simulink model "V2_Modell_RLC"  (R2022a)
settings: Solver=ode3  StartTime=0.0  StopTime=Zeit(end)  FixedStep=0.000001  RelTol=1e-3
values from neighbouring files (symbols this model uses):
  den = [(C*L*R_d*R_v) (R_d*L + R_v*L + R_v*R_d*R_L*C) (R_d*R_L + R_v*R_L + R_v*R_d)]    [V2_Parameter_RLC_gemessen.m]    (also in V2_Parameter_RLC_nominal.m; V2_Parameter_RLC_optimiert.m)
  num = [(R_d * L) (R_d * R_L)]    [V2_Parameter_RLC_gemessen.m]    (also in V2_Parameter_RLC_nominal.m; V2_Parameter_RLC_optimiert.m)
settings Model: Creator=bornkessel  LastModifiedBy=bornkessel

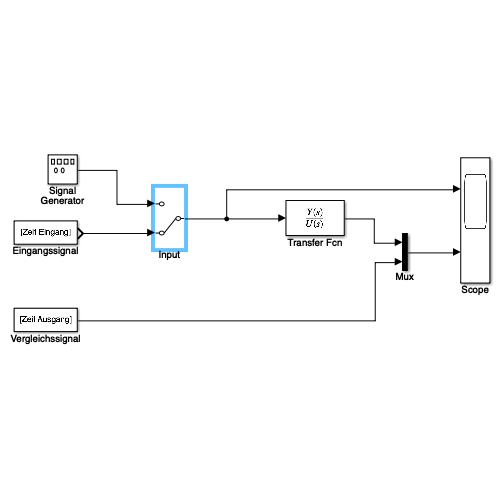
[thumbnail: Simulink's stored preview of the top-level diagram]
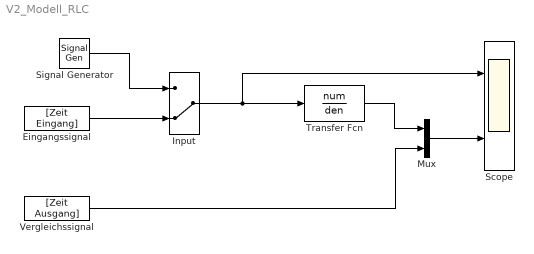
== system V2_Modell_RLC ==
  Eingangssignal : FromWorkspace  VariableName=[Zeit Eingang]
  Input : ManualSwitch  CurrentSetting=0
  Mux : Mux  Inputs=2
  Scope : Scope  NumInputPorts=2
  Signal Generator : SignalGenerator  WaveForm=square  Amplitude=5  Frequency=10
  Transfer Fcn : TransferFcn  Numerator=num  Denominator=den
  Vergleichssignal : FromWorkspace  VariableName=[Zeit Ausgang]
  wires:
  Eingangssignal/1 -> Input/2
  Input/1 -> Scope/1, Transfer Fcn/1
  Signal Generator/1 -> Input/1
  Mux/1 -> Scope/2
  Transfer Fcn/1 -> Mux/1
  Vergleichssignal/1 -> Mux/2
